simulink model "non_linear_dynamics_system"  (R2022b)
settings: Solver=VariableStepAuto  StartTime=0.0  StopTime=10.0  RelTol=1e-3
undefined symbols (not defined in the file): c, f, g, J, Kb, Km, Ku, L, M, Nr, r, Ra
settings Model: Creator=X1  LastModifiedBy=X1

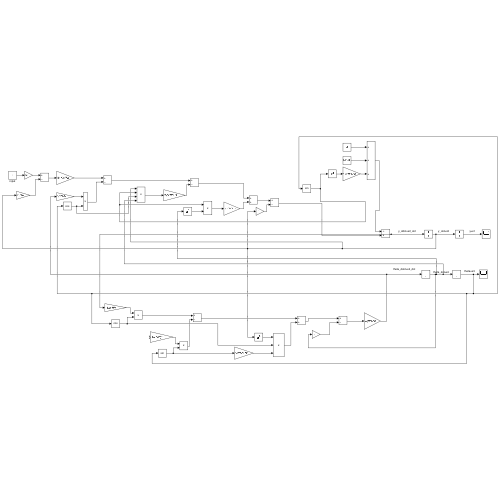
[thumbnail: Simulink's stored preview of the top-level diagram]
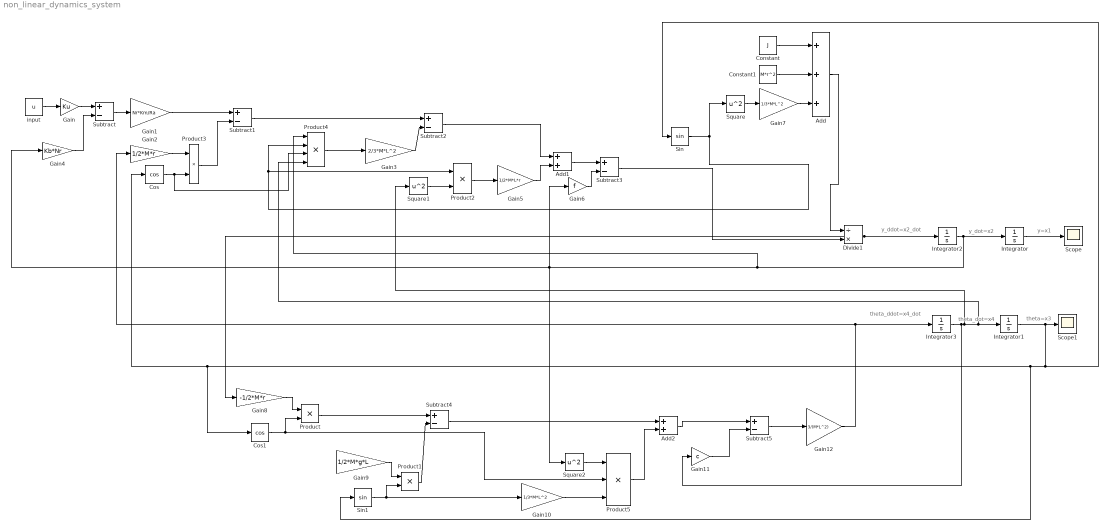
== system non_linear_dynamics_system ==
  note: theta_ddot=x4_dot
  note: y_ddot=x2_dot
  note: y_dot=x2
  note: y=x1
  note: theta_dot=x4
  note: theta=x3
  Add : Sum  Inputs=+++
  Add1 : Sum
  Add2 : Sum
  Constant : Constant  Value=J
  Constant1 : Constant  Value=M*r^2
  Cos : Trigonometry  Operator=cos
  Cos1 : Trigonometry  Operator=cos
  Divide1 : Product  Inputs=/*
  Gain : Gain  Gain=Ku
  Gain1 : Gain  Gain=Nr*Km/Ra
  Gain10 : Gain  Gain=1/3*M*L^2
  Gain11 : Gain  Gain=c
  Gain12 : Gain  Gain=3/(M*L^2)
  Gain2 : Gain  Gain=1/2*M*r
  Gain3 : Gain  Gain=2/3*M*L^2
  Gain4 : Gain  Gain=Kb*Nr
  Gain5 : Gain  Gain=1/2*M*L*r
  Gain6 : Gain  Gain=f
  Gain7 : Gain  Gain=1/3*M*L^2
  Gain8 : Gain  Gain=-1/2*M*r
  Gain9 : Gain  Gain=1/2*M*g*L
  Integrator{,1..3} (4 alike) : Integrator
  Product{,1..3} (4 alike) : Product
  Product4 : Product  Inputs=4
  Product5 : Product  Inputs=3
  Scope : Scope
  Scope1 : Scope
  Sin : Trigonometry
  Sin1 : Trigonometry
  Square : Math  Operator=square
  Square1 : Math  Operator=square
  Square2 : Math  Operator=square
  Subtract{,1..5} (6 alike) : Sum  Inputs=+-
  input : Constant  Value=u
  wires:
  Integrator/1 -> Scope/1
  Integrator2/1 -> Gain4/1, Square2/1, Gain6/1, Product4/1, Integrator/1
  Integrator3/1 -> Product4/4, Integrator1/1, Square1/1, Gain11/1
  Integrator1/1 -> Sin/1, Sin1/1, Cos1/1, Cos/1, Scope1/1
  Sin/1 -> Square/1, Product4/2, Product2/1
  Square/1 -> Gain7/1
  Constant/1 -> Add/1
  Constant1/1 -> Add/2
  input/1 -> Gain/1
  Gain/1 -> Subtract/1
  Subtract/1 -> Gain1/1
  Gain1/1 -> Subtract1/1
  Gain2/1 -> Product3/1
  Cos/1 -> Product4/3, Product3/2
  Product3/1 -> Subtract1/2
  Product4/1 -> Gain3/1
  Subtract1/1 -> Subtract2/1
  Gain3/1 -> Subtract2/2
  Gain4/1 -> Subtract/2
  Square1/1 -> Product2/2
  Product2/1 -> Gain5/1
  Subtract2/1 -> Add1/1
  Gain5/1 -> Add1/2
  Add1/1 -> Subtract3/1
  Gain6/1 -> Subtract3/2
  Gain7/1 -> Add/3
  Divide1/1 -> Integrator2/1, Gain8/1
  Subtract3/1 -> Divide1/2
  Add/1 -> Divide1/1
  Gain12/1 -> Integrator3/1, Gain2/1
  Gain8/1 -> Product/1
  Cos1/1 -> Product5/2, Product/2
  Product/1 -> Subtract4/1
  Gain9/1 -> Product1/1
  Sin1/1 -> Gain10/1, Product1/2
  Product1/1 -> Subtract4/2
  Subtract4/1 -> Add2/1
  Gain10/1 -> Product5/3
  Square2/1 -> Product5/1
  Product5/1 -> Add2/2
  Add2/1 -> Subtract5/1
  Gain11/1 -> Subtract5/2
  Subtract5/1 -> Gain12/1
